simulink model "romOperator"  (Simulink 8.1)
settings: Solver=ode45  StartTime=0.0  StopTime=inf  RelTol=1e-3
settings Model: Creator=eiseles  LastModifiedBy=eiseles
settings DataIOCC: SignalLoggingSaveFormat=Dataset
settings OptimizationCC: ExpressionDepthLimit=128
settings DebuggingCC: FcnCallInpInsideContextMsg=EnableAllAsError
settings GRTTargetCC: CombineOutputUpdateFcns=on  GRTInterface=off

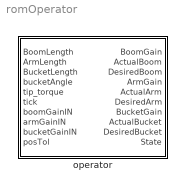
== system romOperator ==
  operator : Subsystem

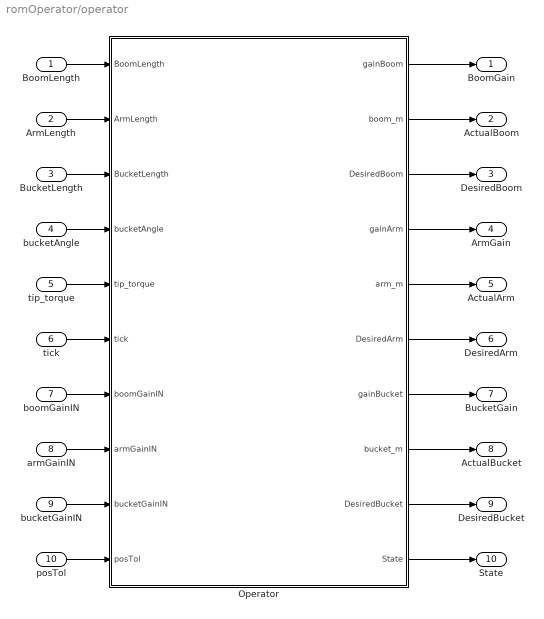
== system romOperator/operator ==
  BoomLength : Inport
  ArmLength : Inport  Port=2
  BucketLength : Inport  Port=3
  bucketAngle : Inport  Port=4
  tip_torque : Inport  Port=5
  tick : Inport  Port=6
  boomGainIN : Inport  Port=7
  armGainIN : Inport  Port=8
  bucketGainIN : Inport  Port=9
  posTol : Inport  Port=10
  Operator : Stateflow chart  TreatAsAtomicUnit=on
  BoomGain : Outport
  ActualBoom : Outport  Port=2
  DesiredBoom : Outport  Port=3
  ArmGain : Outport  Port=4
  ActualArm : Outport  Port=5
  DesiredArm : Outport  Port=6
  BucketGain : Outport  Port=7
  ActualBucket : Outport  Port=8
  DesiredBucket : Outport  Port=9
  State : Outport  Port=10
  wires:
  bucketAngle/1 -> Operator/4(bucketAngle)
  BoomLength/1 -> Operator/1(BoomLength)
  BucketLength/1 -> Operator/3(BucketLength)
  tip_torque/1 -> Operator/5(tip_torque)
  ArmLength/1 -> Operator/2(ArmLength)
  Operator/2(boom_m) -> ActualBoom/1
  Operator/3(DesiredBoom) -> DesiredBoom/1
  Operator/4(gainArm) -> ArmGain/1
  Operator/1(gainBoom) -> BoomGain/1
  Operator/6(DesiredArm) -> DesiredArm/1
  Operator/7(gainBucket) -> BucketGain/1
  Operator/9(DesiredBucket) -> DesiredBucket/1
  Operator/5(arm_m) -> ActualArm/1
  Operator/8(bucket_m) -> ActualBucket/1
  tick/1 -> Operator/6(tick)
  Operator/10(State) -> State/1
  boomGainIN/1 -> Operator/7(boomGainIN)
  armGainIN/1 -> Operator/8(armGainIN)
  bucketGainIN/1 -> Operator/9(bucketGainIN)
  posTol/1 -> Operator/10(posTol)

== stateflow chart operator/Operator ==
  state Lifting
    entry: State= 2;
    boom_m = BoomLength;
    arm_m = ArmLength;
    bucket_m = -bucketAngle;
    DesiredBoom = .95;
    DesiredArm = .95;
    DesiredBucket = levelBucket;
    gainBoom = boomGainIN;
    gainArm = armGainIN;
    gainBucket = bucketGainIN;
    during:boom_m = BoomLength;
    arm_m = ArmLength;
    bucket_m = -bucketAngle;
  state Digging
    en: State = 11;
    bucket_m = -bucketAngle;
    DesiredBucket = 0;
    DesiredArm = .95;
    du:
    boom_m = BoomLength;
    arm_m = ArmLength;
    bucket_m = -bucketAngle;
  state dug
    en: State = 12;
  state Extended
    entry: State= 6;
  state Dumped
    en: State = 8;
    en,du: boom_m = BoomLength;
    arm_m = ArmLength;
    bucket_m = BucketLength;
  state Decending
    en: State = 9;
    DesiredBoom = .05;
    du:
    boom_m = BoomLength;
    arm_m = ArmLength;
    bucket_m = BucketLength;
  state intial
    en: State = 0;
    DesiredBoom = BoomLength;
    DesiredArm = ArmLength;
    DesiredBucket = BucketLength;
    gainBoom = boomGainIN;
    gainArm = armGainIN;
    gainBucket = bucketGainIN;
    during:boom_m = BoomLength;
    arm_m = ArmLength;
    bucket_m = BucketLength;
  state Lifted
    entry: State= 3;
  state bucketCyl_maxed
    entry: State = 5;
    DesiredBucket = .05;
    boom_m = BoomLength;
    arm_m = ArmLength;
    bucket_m = BucketLength;
    during:boom_m = BoomLength;
    arm_m = ArmLength;
    bucket_m = BucketLength;
  state Decended
    en: State = 10;
  state capturing
    en: State = 13;
    bucket_m = BucketLength;
    DesiredBucket = .95;
    du:
    boom_m = BoomLength;
    arm_m = ArmLength;
    bucket_m = BucketLength;
  state Extending
    entry: State= 4;
    boom_m = BoomLength;
    arm_m = ArmLength;
    bucket_m = -bucketAngle;
    DesiredBoom = .95;
    DesiredArm = .05;
    DesiredBucket = .05;
    gainArm = armGainIN*.3;
    during:boom_m = BoomLength;
    arm_m = ArmLength;
    bucket_m = -bucketAngle;
  state captured
    entry: State= 1;
    boom_m = BoomLength;
    arm_m = ArmLength;
    bucket_m = -bucketAngle;
    DesiredBoom = .05;
    DesiredArm = .95;
    DesiredBucket = levelBucket;
    during:boom_m = BoomLength;
    arm_m = ArmLength;
    bucket_m = -bucketAngle;
  state Dumping
    entry: State= 7;
    boom_m = BoomLength;
    arm_m = ArmLength;
    bucket_m = BucketLength;
    DesiredBoom = .95;
    DesiredArm = .01;
    DesiredBucket = .05;
    during: boom_m = BoomLength;
    arm_m = ArmLength;
    bucket_m = BucketLength;
  Extending -> bucketCyl_maxed [order 3] : [BucketLength>=.95]
  Lifted -> Extending : [tick==1]
  bucketCyl_maxed -> Extended : [arm_m<=DesiredArm + posTol]
  Lifting -> Lifted : [boom_m>=DesiredBoom-posTol &&...
      |  boom_m<= DesiredBoom + posTol &&...
      |  arm_m >= DesiredArm-posTol && ...
      |  arm_m <= DesiredArm + posTol]
  Extending -> Extended [order 1] : [arm_m<=DesiredArm+posTol ]
  Extending -> Dumping [order 2] : [-bucketAngle<=.6]
  Extended -> Dumping : [tick==1]
  intial -> Lifting : [DesiredBoom - .01 >= boom_m <= DesiredBoom +.01 &&...
      |  DesiredArm - .01    >= arm_m <= DesiredArm+.01 &&...
      |  DesiredBucket-.01 >= bucket_m <= DesiredBucket+.01]
  captured -> Lifting : [tick==1]
  Dumping -> Dumped : [bucket_m<=DesiredBucket + posTol]
  (default) -> intial
  capturing -> captured : [bucket_m>=DesiredBucket-posTol]
  Dumped -> Decending : [tick==1]
  Decending -> Decended : [boom_m<=DesiredBoom+posTol]
  Decended -> Digging : [tick==1]
  Digging -> dug : [arm_m>= DesiredArm-posTol]
  dug -> capturing : [tick==1]
  data: gainBoom output double =1; boom_m output double; DesiredBoom output double; gainArm output double =1; arm_m output double; DesiredArm output double; BoomLength input double; ArmLength input double; BucketLength input double; bucketAngle input double; gainBucket output double =1; bucket_m output double; DesiredBucket output double; tip_torque input double; max_torque local double =1e5; tick input double; State output double; FinalArm local double; levelBucket local double =1.8; boomGainIN input double; armGainIN input double; bucketGainIN input double; posTol input double
